simulink model "Project_discrete_sim"  (R2016b)
settings: Solver=FixedStepAuto  StartTime=0.0  StopTime=1  FixedStep=.001  RelTol=1e-3
settings Model: Creator=hp  LastModifiedBy=anshu
settings SolverCC: AutoInsertRateTranBlk=on

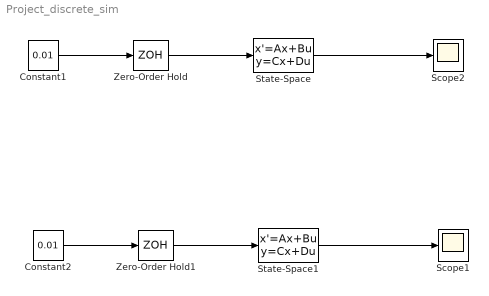
== system Project_discrete_sim ==
  Constant1 : Constant  Description=Simulation Model Input  Value=0.01  SampleTime=.005
      settings: AttributesFormatString=|
      | Simulation Model
      | Input-Constant
      | Sample time 0.005
  Constant2 : Constant  Description=Simulation Model Input  Value=0.01  SampleTime=.03
      settings: AttributesFormatString=|
      | Simulation Model
      | Input-Constant
      | Sample time 0.03
  Scope1 : Scope
      settings: Description=Output for constant Input
      settings: AttributesFormatString=|
      | Output ZOH
      | constant Input
  Scope2 : Scope
      settings: Description=Output for constant Input
      settings: AttributesFormatString=|
      | Output ZOH
      | constant Input
  State-Space : StateSpace  Tag=Ballbot  Description=|  A=|  B=|  C=[1, 0, 0, 0; 0, 0, 1, 0]  D=[0; 0]  X0=0
      A=|
      | [ 0, 1.0000, 0, 0; 0, -0.6698, -477.3945, 0; 0, 0, 0, 1.0000;
      | 0, 0.1477,  122.6790, 0]
      B=|
      | [0;
      | 69.7518;
      | 0;
      | -15.2579]
      Description=|
      | State space representation of Ballbot
      | Constant Input
      settings: AttributesFormatString=|
      | State space representation of Ballbot
      | Constant Input
  State-Space1 : StateSpace  Tag=Ballbot  Description=|  A=|  B=|  C=[1, 0, 0, 0; 0, 0, 1, 0]  D=[0; 0]  X0=0
      A=|
      | [ 0, 1.0000, 0, 0; 0, -0.6698, -477.3945, 0; 0, 0, 0, 1.0000;
      | 0, 0.1477,  122.6790, 0]
      B=|
      | [0;
      | 69.7518;
      | 0;
      | -15.2579]
      Description=|
      | State space representation of Ballbot
      | Constant Input
      settings: AttributesFormatString=|
      | State space representation of Ballbot
      | Constant Input
  Zero-Order Hold : ZeroOrderHold  SampleTime=.005
  Zero-Order Hold1 : ZeroOrderHold  SampleTime=.03
  wires:
  Constant1/1 -> Zero-Order Hold/1
  Zero-Order Hold/1 -> State-Space/1
  State-Space/1 -> Scope2/1
  Constant2/1 -> Zero-Order Hold1/1
  Zero-Order Hold1/1 -> State-Space1/1
  State-Space1/1 -> Scope1/1
